simulink model "Project3Week1_notireslip"  (R2024b)
settings: Solver=VariableStepAuto  StartTime=0.0  StopTime=765  RelTol=1e-3
values from neighbouring files (symbols this model uses):
  ad = 2.25    [Project3Week1.m]
  cd = 0.34    [Project3Week1.m]
  gratio = 2    [Project3Week1.m]
  i_gear_i = 0.5    [Project3Week1.m]
  ipt = 10    [Project3Week1.m]
  iw = 9    [Project3Week1.m]
  kd = .005    (= 0.005)    [Project3Week1.m]
  ki = .02    (= 0.02)    [Project3Week1.m]
  kp = 0.0075    [Project3Week1.m]
  l_time = l_time(2:end)    [Project3Week1.m]
  l_vel = l_vel(2:end) * 0.44704    [Project3Week1.m]
  o_gear_i = 0.7    [Project3Week1.m]
  rho = 1.293    [Project3Week1.m]
  rw = 0.48/2    (= 0.24)    [Project3Week1.m]
  tau_brakes = 1500    [Project3Week1.m]
  tau_motor = 800    [Project3Week1.m]
  vm = 1600    [Project3Week1.m]
settings Model: Creator=btagl  LastModifiedBy=btagl

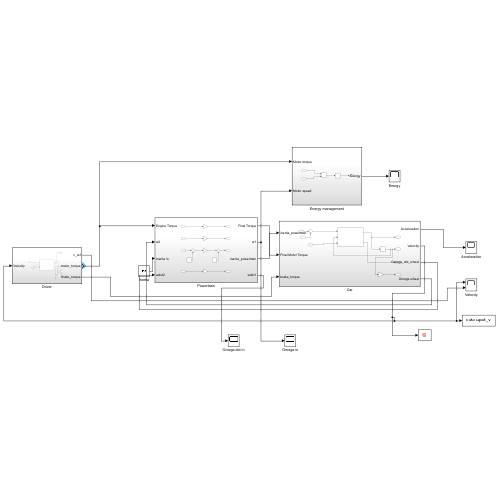
[thumbnail: Simulink's stored preview of the top-level diagram]
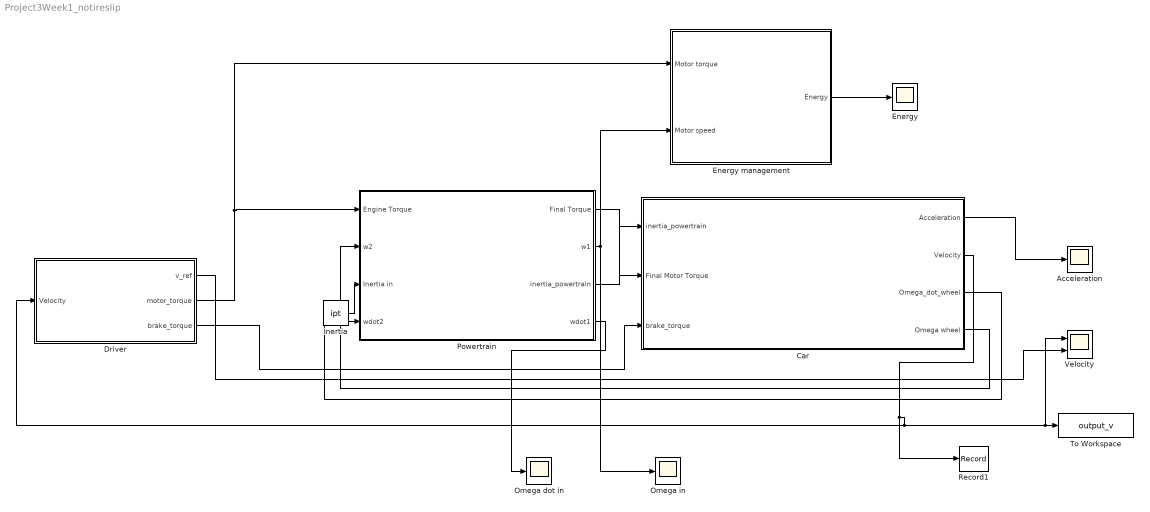
== system Project3Week1_notireslip ==
  Acceleration : Scope
  Car : Subsystem
  Driver : Subsystem
  Energy : Scope
  Energy management : Subsystem
  Inertia : Constant  Value=ipt
  Omega dot in : Scope
  Omega in : Scope
  Powertrain : Subsystem
  Record1 : Record  VariableName=actual_v  RecordToWorkspace=on  FileSettingsInternal="{\"entries\":[{\"content\":{\"excelSettings\":{\"content\":{},\"type\":\"Streamout.ExcelSettings\"}},\"type\":\"Streamout.FileSettingStorage\",\"uuid\":\"\"}],\"packageUris\":[\"http:\\/\\/schema.mathworks.com\\/mf0\\/streamout_blocks\\/R2020a\"],\"version\":\"1.0\"}"  SignalsInternal="{\"entries\":[{\"content\":{\"signals\":[{\"content\":{\"blockPath\":[],\"dimensions\":[1],\"domain\":\"\",\"lineColor\":\"#4dbeee\",\"lineWidth\":2,\"plots\":[ 1 ],\"port\":1,\"sid\":[\"\"],\"signalID\":1,\"signalName\":\"Car:2\"},\"type\":\"RecordBlkView.Signal\",\"uuid\":\"\"}]},\"type\":\"RecordBlkView.InputSignals\",\"uuid\":\"\"}],\"packageUris\":[\"http:\\/\\/schema.mathworks.com\\/mf0\\/streamout_blocks\\/R2020a\"],\"version\":\"1.0\"}"  VisualizationBindings="{\"sparklinesplugin\":{\"info\":[{\"bindingParametersList\":[],\"subplotID\":1}]}}"
  To Workspace : ToWorkspace  VariableName=output_v  SampleTime=-1
  Velocity : Scope  NumInputPorts=2
  wires:
  Car/2(Velocity) -> Velocity/1, To Workspace/1, Driver/1(Velocity), Record1/1
  Car/1(Acceleration) -> Acceleration/1
  Driver/1(v_ref) -> Velocity/2
  Powertrain/3(inertia_powertrain) -> Car/1(inertia_powertrain)
  Inertia/1 -> Powertrain/3(Inertia in)
  Car/4(Omega wheel) -> Powertrain/2(w2)
  Powertrain/2(w1) -> Omega in/1, Energy management/2(Motor speed)
  Powertrain/4(wdot1) -> Omega dot in/1
  Car/3(Omega_dot_wheel) -> Powertrain/4(wdot2)
  Energy management/1(Energy) -> Energy/1
  Driver/2(motor_torque) -> Energy management/1(Motor torque), Powertrain/1(Engine Torque)
  Powertrain/1(Final Torque) -> Car/2(Final Motor Torque)
  Driver/3(brake_torque) -> Car/3(brake_torque)

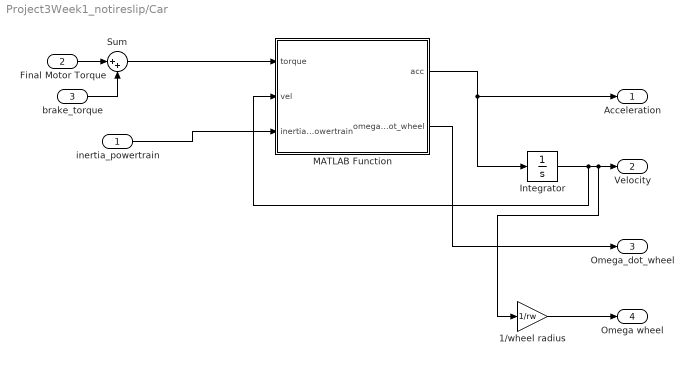
== system Project3Week1_notireslip/Car ==
  inertia_powertrain : Inport
  Final Motor Torque : Inport  Port=2
  brake_torque : Inport  Port=3
  1/wheel radius : Gain  Gain=1/rw
  Integrator : Integrator
  MATLAB Function : MATLAB Function  TreatAsAtomicUnit=on
  Sum : Sum  Inputs=|++
  Acceleration : Outport
  Velocity : Outport  Port=2
  Omega_dot_wheel : Outport  Port=3
  Omega wheel : Outport  Port=4
  wires:
  Sum/1 -> MATLAB Function/1(torque)
  MATLAB Function/1(acc) -> Integrator/1, Acceleration/1
  Integrator/1 -> MATLAB Function/2(vel), 1/wheel radius/1, Velocity/1
  inertia_powertrain/1 -> MATLAB Function/3(inertia_powertrain)
  MATLAB Function/2(omega_dot_wheel) -> Omega_dot_wheel/1
  1/wheel radius/1 -> Omega wheel/1
  Final Motor Torque/1 -> Sum/1
  brake_torque/1 -> Sum/2

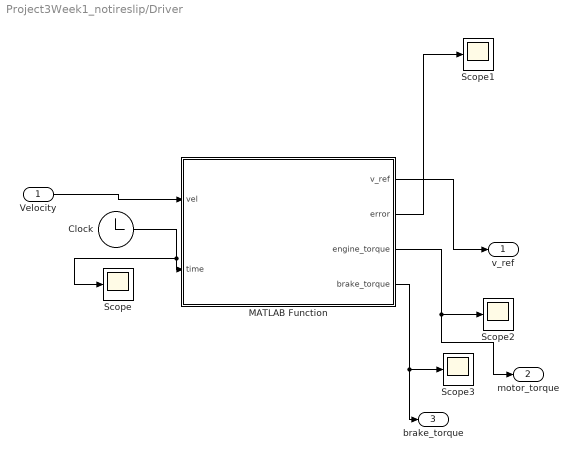
== system Project3Week1_notireslip/Driver ==
  Velocity : Inport
  Clock : Clock
  MATLAB Function : MATLAB Function  TreatAsAtomicUnit=on
  Scope{,1..3} (4 alike) : Scope
  v_ref : Outport
  motor_torque : Outport  Port=2
  brake_torque : Outport  Port=3
  wires:
  Velocity/1 -> MATLAB Function/1(vel)
  Clock/1 -> Scope/1, MATLAB Function/2(time)
  MATLAB Function/1(v_ref) -> v_ref/1
  MATLAB Function/2(error) -> Scope1/1
  MATLAB Function/3(engine_torque) -> motor_torque/1, Scope2/1
  MATLAB Function/4(brake_torque) -> brake_torque/1, Scope3/1

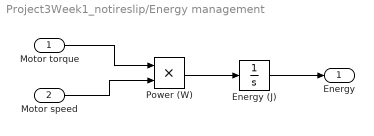
== system Project3Week1_notireslip/Energy management ==
  Motor torque : Inport
  Motor speed : Inport  Port=2
  Energy (J) : Integrator
  Power (W) : Product
  Energy : Outport
  wires:
  Motor torque/1 -> Power (W)/1
  Motor speed/1 -> Power (W)/2
  Power (W)/1 -> Energy (J)/1
  Energy (J)/1 -> Energy/1

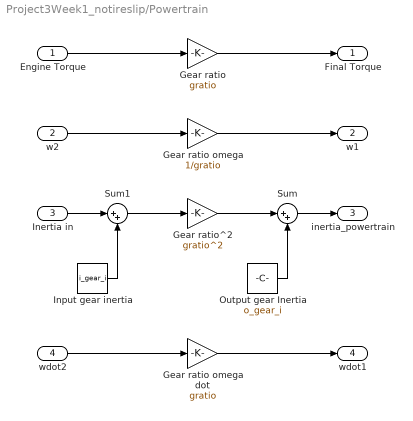
== system Project3Week1_notireslip/Powertrain ==
  Engine Torque : Inport
  w2 : Inport  Port=2
  Inertia in : Inport  Port=3
  wdot2 : Inport  Port=4
  Gear ratio : Gain  Gain=gratio
  Gear ratio omega : Gain  Gain=1/gratio
  Gear ratio omega dot : Gain  Gain=gratio
  Gear ratio^2 : Gain  Gain=gratio^2
  Input gear inertia : Constant  Value=i_gear_i
  Output gear Inertia : Constant  Value=o_gear_i
  Sum : Sum  Inputs=|++
  Sum1 : Sum  Inputs=|++
  Final Torque : Outport
  w1 : Outport  Port=2
  inertia_powertrain : Outport  Port=3
  wdot1 : Outport  Port=4
  wires:
  Engine Torque/1 -> Gear ratio/1
  Gear ratio/1 -> Final Torque/1
  Gear ratio omega/1 -> w1/1
  w2/1 -> Gear ratio omega/1
  Input gear inertia/1 -> Sum1/2
  Inertia in/1 -> Sum1/1
  Sum1/1 -> Gear ratio^2/1
  Output gear Inertia/1 -> Sum/2
  Gear ratio^2/1 -> Sum/1
  Sum/1 -> inertia_powertrain/1
  Gear ratio omega dot/1 -> wdot1/1
  wdot2/1 -> Gear ratio omega dot/1

== matlab function Project3Week1_notireslip/Driver/MATLAB Function ==
  settings: updateMethod=DISCRETE  sampleTime=0.001
  data: vel input; tau_motor parameter; time input; l_time parameter; l_vel parameter; v_ref output; error output; kp parameter; ki parameter; kd parameter; tau_brakes parameter; engine_torque output; brake_torque output
function [v_ref,error,engine_torque,brake_torque]= driver_model(vel, tau_motor,time,l_time,l_vel,kp, ki, kd, tau_brakes)

    % Persistent variables for integral and previous error
    persistent integral_error prev_error;
    if isempty(integral_error)
        integral_error = 0;
        prev_error = 0;
    end
    
    % Compute reference velocity
    v_ref = interp1(l_time, l_vel, time, 'linear', 'extrap');    
    error = v_ref - vel;
    
    % PID Controller
    integral_error = integral_error + error;
    derivative_error = error - prev_error;
    prev_error = error;

    % Compute control output (alpha_driver)
    alpha_driver = kp * error + ki * integral_error + kd * derivative_error;

    % Limit alpha_driver to range [-1, 1]
    alpha_driver = max(-1, min(1, alpha_driver));

    % Compute torque
    if alpha_driver >= 0
        engine_torque=alpha_driver*tau_motor;
        brake_torque=0;
    else
        engine_torque=0;
        brake_torque=alpha_driver*tau_brakes;
    end
end

== matlab function Project3Week1_notireslip/Car/MATLAB Function ==
  data: acc output; torque input; iw parameter; rw parameter; vm parameter; cd parameter; vel input; ad parameter; rho parameter; inertia_powertrain input; omega_dot_wheel output
function [acc, omega_dot_wheel] = fcn(torque, iw, rw, vm, cd,vel,ad,rho, inertia_powertrain)

fdrag=0.5*(rho*ad*cd*vel^2);
meq=((inertia_powertrain+iw)/rw^2)+vm;
fx=(torque/rw)-fdrag;
acc=(fx/meq);
omega_dot_wheel=acc/rw; %rad/s^2 angular acceleration
